simulink model "motor"  (R2022b)
settings: Solver=VariableStepAuto  StartTime=0.0  StopTime=10.0  RelTol=1e-3
settings Model: Creator=fabian  LastModifiedBy=fabian

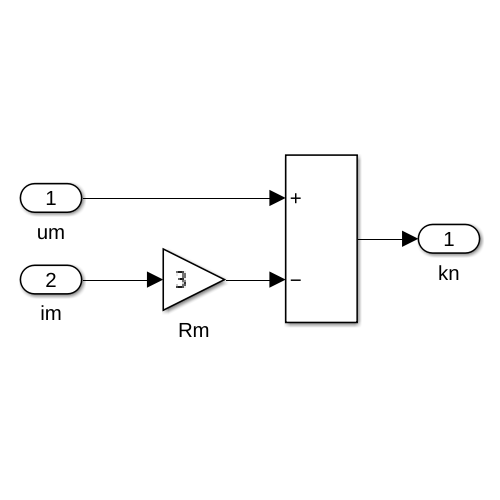
[thumbnail: Simulink's stored preview of the top-level diagram]
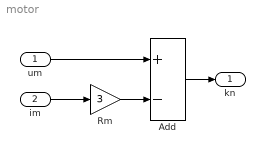
== system motor ==
  um : Inport
  im : Inport  Port=2
  Add : Sum  Inputs=+-
  Rm : Gain  Gain=3
  kn : Outport
  wires:
  im/1 -> Rm/1
  Rm/1 -> Add/2
  um/1 -> Add/1
  Add/1 -> kn/1
